simulink model "on_off_thruster"  (R2015b)
settings: Solver=VariableStepAuto  StartTime=0.0  StopTime=stop_time  RelTol=1e-9
undefined symbols (not defined in the file): alpha_0, alpha_1, I_y, omega_y_0, Q_0, tau_y, theta_0
settings Model: Creator=Krunal's PC  LastModifiedBy=Krunal's PC

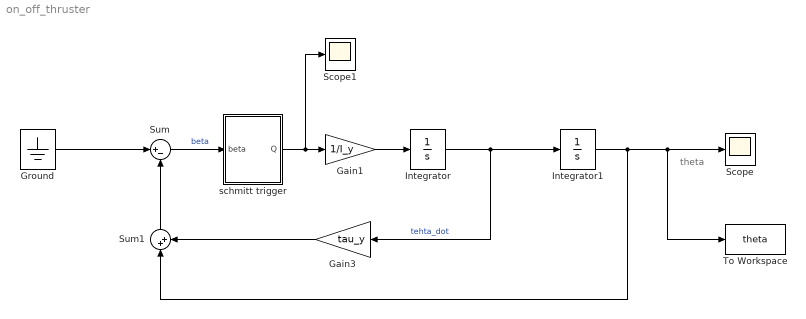
== system on_off_thruster ==
  note: theta
  Gain1 : Gain  Gain=1/I_y
  Gain3 : Gain  Gain=tau_y
  Ground : Ground
  Integrator : Integrator  InitialCondition=omega_y_0
  Integrator1 : Integrator  InitialCondition=theta_0
  Scope : Scope
  Scope1 : Scope
  Sum : Sum  Inputs=|+-
  Sum1 : Sum  Inputs=|++
  To Workspace : ToWorkspace  VariableName=theta  SampleTime=-1
  schmitt trigger : Subsystem
  wires:
  Gain1/1 -> Integrator/1
  Integrator/1 -> Gain3/1, Integrator1/1  "tehta_dot"
  Integrator1/1 -> Sum1/1, To Workspace/1, Scope/1
  Ground/1 -> Sum/1
  Gain3/1 -> Sum1/2
  Sum1/1 -> Sum/2
  Sum/1 -> schmitt trigger/1(beta)  "beta"
  schmitt trigger/1(Q) -> Scope1/1, Gain1/1

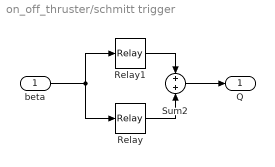
== system on_off_thruster/schmitt trigger ==
  beta : Inport
  Relay : Relay  OnSwitchValue=alpha_1  OffSwitchValue=alpha_0  OnOutputValue=Q_0
  Relay1 : Relay  OnSwitchValue=-alpha_0  OffSwitchValue=-alpha_1  OnOutputValue=0  OffOutputValue=-Q_0
  Sum2 : Sum  Inputs=+|+
  Q : Outport
  wires:
  Relay1/1 -> Sum2/1
  beta/1 -> Relay/1, Relay1/1
  Relay/1 -> Sum2/2
  Sum2/1 -> Q/1
